simulink model "control2"  (R2020b)
settings: Solver=FixedStepAuto  StartTime=0.0  StopTime=9  FixedStep=1e-2  RelTol=1e-3
libraries: pid_lib x1
settings Model: Creator=angello  LastModifiedBy=angello

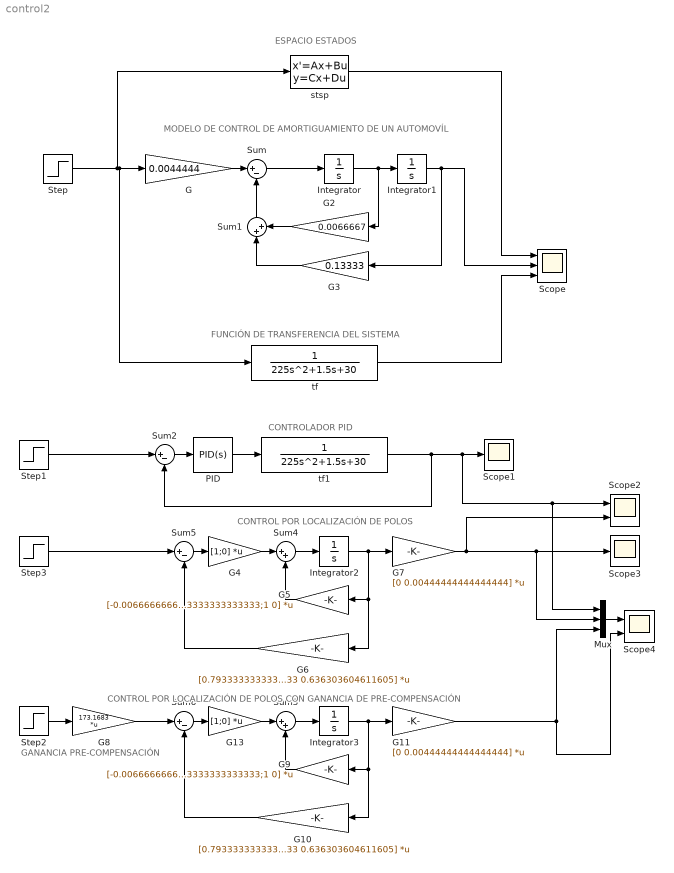
== system control2 ==
  note: GANANCIA PRE-COMPENSACIÓN
  note: ESPACIO ESTADOS
  note: MODELO DE CONTROL DE AMORTIGUAMIENTO DE UN AUTOMOVÍL
  note: FUNCIÓN DE TRANSFERENCIA DEL SISTEMA
  note: CONTROLADOR PID
  note: CONTROL POR LOCALIZACIÓN DE POLOS
  note: CONTROL POR LOCALIZACIÓN DE POLOS CON GANANCIA DE PRE-COMPENSACIÓN
  G : Gain  Gain=0.0044444
  G10 : Gain  Gain=[0.793333333333333 0.636303604611605]  Multiplication=Matrix(K*u)
  G11 : Gain  Gain=[0 0.00444444444444444]  Multiplication=Matrix(K*u)
  G13 : Gain  Gain=[1;0]  Multiplication=Matrix(K*u)
  G2 : Gain  Gain=0.0066667
  G3 : Gain  Gain=0.13333
  G4 : Gain  Gain=[1;0]  Multiplication=Matrix(K*u)
  G5 : Gain  Gain=[-0.00666666666666667 -0.133333333333333;1 0]  Multiplication=Matrix(K*u)
  G6 : Gain  Gain=[0.793333333333333 0.636303604611605]  Multiplication=Matrix(K*u)
  G7 : Gain  Gain=[0 0.00444444444444444]  Multiplication=Matrix(K*u)
  G8 : Gain  Gain=173.1683  Multiplication=Matrix(K*u)
  G9 : Gain  Gain=[-0.00666666666666667 -0.133333333333333;1 0]  Multiplication=Matrix(K*u)
  Integrator{,1..3} (4 alike) : Integrator
  Mux : Mux  Inputs=3
  PID : pid_lib/PID Controller  Controller=PID  Form=Parallel  TimeDomain=Continuous-time  UseExternalTs=off  SampleTime=-1  IntegratorMethod=Forward Euler  FilterMethod=Forward Euler  ControllerParametersSource=internal  P=863.1683  I=692.6732  D=1078.5  UseFilter=on  N=100  TunerSelectOption=Transfer Function Based (PID Tuner App)  InitialConditionSource=internal  InitialConditionForIntegrator=0  InitialConditionForFilter=0  DifferentiatorICPrevScaledInput=0  ExternalReset=none  TrackingMode=off  Kt=1  LimitOutput=off  SatLimitsSource=internal  UpperSaturationLimit=inf  LowerSaturationLimit=-inf  LinearizeAsGain=on  AntiWindupMode=none  Kb=1  POutMin=[]  POutMax=[]  IOutMin=[]  IOutMax=[]  DOutMin=[]  DOutMax=[]  NOutMin=[]  NOutMax=[]  SumOutMin=[]  SumOutMax=[]  SaturationOutMin=[]  SaturationOutMax=[]  PParamMin=[]  PParamMax=[]  IParamMin=[]  IParamMax=[]  DParamMin=[]  DParamMax=[]  NParamMin=[]  NParamMax=[]  KbParamMin=[]  KbParamMax=[]  KtParamMin=[]  KtParamMax=[]  KbOutMin=[]  KbOutMax=[]  KtOutMin=[]  KtOutMax=[]  IntegratorOutMin=[]  IntegratorOutMax=[]  FilterOutMin=[]  FilterOutMax=[]  SumI1OutMin=[]  SumI1OutMax=[]  SumI2OutMin=[]  SumI2OutMax=[]  SumI3OutMin=[]  SumI3OutMax=[]  SumI4OutMin=[]  SumI4OutMax=[]  SumDOutMin=[]  SumDOutMax=[]  DifferentiatorOutMin=[]  DifferentiatorOutMax=[]  FilterDiffOutCoefMin=[]  FilterDiffOutCoefMax=[]  ReciprocalOutMin=[]  ReciprocalOutMax=[]  SumDenOutMin=[]  SumDenOutMax=[]  SumNumOutMin=[]  SumNumOutMax=[]  DivideOutMin=[]  DivideOutMax=[]  UdiffTsProdOutMin=[]  UdiffTsProdOutMax=[]  NTsProdOutMin=[]  NTsProdOutMax=[]  UintegralTsProdOutMin=[]  UintegralTsProdOutMax=[]  UngainTsProdOutMin=[]  UngainTsProdOutMax=[]  IntegratorContinuousStateAttributes=''  IntegratorStateMustResolveToSignalObject=off  IntegratorRTWStateStorageClass=Auto  FilterContinuousStateAttributes=''  FilterStateMustResolveToSignalObject=off  FilterRTWStateStorageClass=Auto  ParallelPVariant=InternalParameters  IdealPVariant=Disabled  IVariant=InternalParameters  DVariant=InternalParameters  IntegratorVariant=Continuous  SatVariant=Disabled  AWVariant=Passthrough  PCopyVariant=Disabled  TRVariant=Disabled  FdbkBlocksVariant=Forward  IdealPFdbkVariant=Disabled  SatFdbkVariant=Disabled  DerivativeFilterVariant=ContFilter  NVariant=InternalParameters  NCopyVariant=Disabled  FilterICVariant=InternalICsFilter  IntegratorICVariant=InternalICs  ExternalResetVariant=Disabled  TRSumVariant=Passthrough  SumFdbkVariant=Disabled  SumVariant=Sum_PID  TsampFilterVariant=InternalTs  TsampNgainVariant=Passthrough  TsampIntegralVariant=Passthrough  ExternalSaturationOutDataTypeStr=Inherit: Same as second input
  Scope : Scope  NumInputPorts=3
  Scope1 : Scope
  Scope2 : Scope  NumInputPorts=2
  Scope3 : Scope
  Scope4 : Scope  NumInputPorts=2
  Step{,1..3} (4 alike) : Step  Time=0  SampleTime=0
  Sum{,2,5..6} (4 alike) : Sum  Inputs=|+-
  Sum1 : Sum  Inputs=|++
  Sum3 : Sum  Inputs=|++
  Sum4 : Sum  Inputs=|++
  stsp : StateSpace  A=[-0.00666666666666667 -0.133333333333333;1 0]  B=[1;0]  C=[0 0.00444444444444444]  D=0  InitialCondition=0
  tf : TransferFcn  Numerator=1  Denominator=[225 1.5 30]
  tf1 : TransferFcn  Numerator=1  Denominator=[225 1.5 30]
  wires:
  Step/1 -> stsp/1, tf/1, G/1
  stsp/1 -> Scope/1
  tf/1 -> Scope/3
  Integrator/1 -> G2/1, Integrator1/1
  G/1 -> Sum/1
  Sum/1 -> Integrator/1
  Sum1/1 -> Sum/2
  G2/1 -> Sum1/2
  G3/1 -> Sum1/1
  Integrator1/1 -> G3/1, Scope/2
  PID/1 -> tf1/1
  tf1/1 -> Sum2/2, Mux/1, Scope2/1, Scope1/1
  Step1/1 -> Sum2/1
  Sum2/1 -> PID/1
  G5/1 -> Sum4/2
  Integrator2/1 -> G7/1, G5/1, G6/1
  Sum4/1 -> Integrator2/1
  G4/1 -> Sum4/1
  Sum5/1 -> G4/1
  G6/1 -> Sum5/2
  G7/1 -> Mux/2, Scope3/1, Scope2/2
  Step2/1 -> G8/1
  G8/1 -> Sum6/1
  G11/1 -> Scope4/2, Mux/3
  G10/1 -> Sum6/2
  Sum6/1 -> G13/1
  G13/1 -> Sum3/1
  Sum3/1 -> Integrator3/1
  Integrator3/1 -> G10/1, G9/1, G11/1
  G9/1 -> Sum3/2
  Step3/1 -> Sum5/1
  Mux/1 -> Scope4/1
